simulink model "Step_8_Gravity_compensationController"  (R2020a)
settings: Solver=VariableStepAuto  StartTime=0.0  StopTime=20  FixedStep=1e-3  RelTol=1e-3
values from neighbouring files (symbols this model uses):
  N = simplify(N,'Seconds',30)    [GetTheRegressorMatrix_step1.m]    (also in Step_1_TheRegressorModel.m)
  s = size(M)    [GetTheRegressorMatrix_step1.m]    (also in Step_1_TheRegressorModel.m)
  Y = sym(zeros(robot.nbDOF,numel(Xhi)))    [GetTheRegressorMatrix_step1.m]    (also in Step_1_TheRegressorModel.m)
  Z = robot.symbolicParameters.Z    [GetTheRegressorMatrix_step1.m]    (also in Step_1_TheRegressorModel.m)
undefined symbols (not defined in the file or in its folder): X
libraries: sm_lib x73, nesl_utility x19
(part 1 of 2)
settings Model: Creator=nnnmmm  LastModifiedBy=nnnmmm
settings ExplorerConfigSet: InternalSimMechanicsExplorerSettings="<ExplorerConfiguration><canonicalview>default</canonicalview><AnimationSetting><BasePlaybackSpeed>1.0</BasePlaybackSpeed><PlaybackSpeedFactor>1.0</PlaybackSpeedFactor></AnimationSetting><TilePanel><TileInfo><Tiles Columns=\"1\" Count=\"1\" Rows=\"1\"><Column Weight=\"1\"/><Row Weight=\"1\"/><Tile Height=\"1\" Width=\"1\" X=\"0\" Y=\"0\"/></Tiles></TileInfo><SceneInfo><SceneViewer><BGColor><R>0.60000002384185791</R><G>0.60000002384185791</G><B>0.60000002384185791</B></BGColor><Camera><DoPerspective>off</DoPerspective><Position><X>-0.071417138481595005</X><Y>-0.953379631042480469</Y><Z>-0.0736574933478599397</Z></Position><Center><X>-0.071417138481595005</X><Y>0.0466203689575195104</Y><Z>-0.0736574933478599397</Z></Center><Up><X>0</X><Y>-0</Y><Z>1</Z></Up><ViewLimDist>1</ViewLimDist><YLim>0.662662160254506083</YLim><XLim>1.08174302415975299</XLim></Camera></SceneViewer></SceneInfo></TilePanel><MechEditorPanel><Cameras/><GfxPanelCameraMap/><VideoCreator><PlaybackSpeedRatio>1.0</PlaybackSpeedRatio><FrameRate>60</FrameRate><VideoFormat>MPEG-4</VideoFormat><FrameSize>auto</FrameSize></VideoCreator></MechEditorPanel></ExplorerConfiguration>"

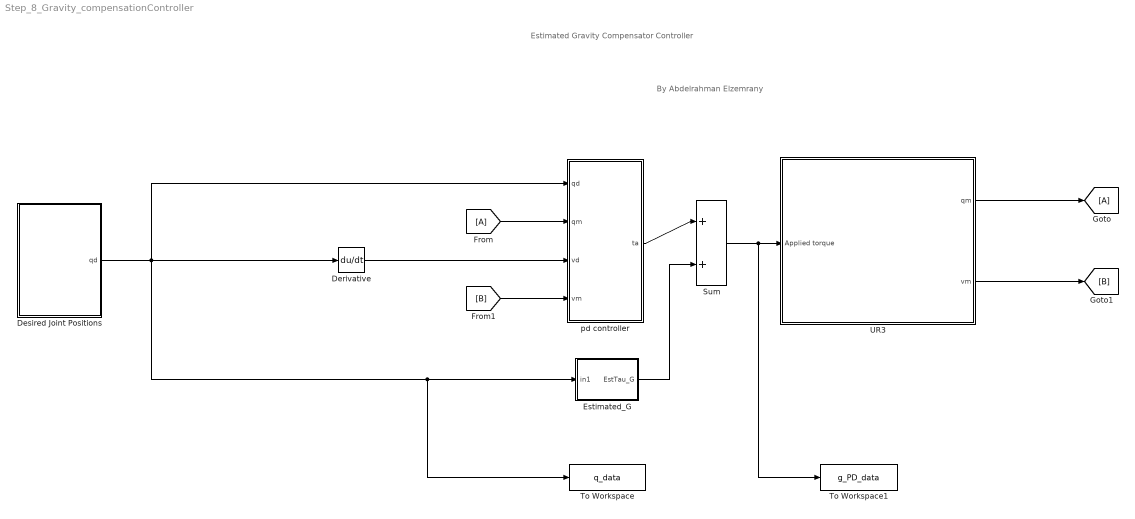
== system Step_8_Gravity_compensationController ==
  note: By Abdelrahman Elzemrany
  note: Estimated Gravity Compensator Controller
  Derivative : Derivative
  Desired Joint Positions : Subsystem
  Estimated_G : MATLAB Function  TreatAsAtomicUnit=on
  Sum : Sum  Inputs=|++
  To Workspace : ToWorkspace  VariableName=q_data  SaveFormat=Timeseries  SampleTime=-1
  To Workspace1 : ToWorkspace  VariableName=g_PD_data  SaveFormat=Timeseries  SampleTime=-1
  UR3 : Subsystem
  pd controller : Subsystem
  wires:
  Desired Joint Positions/1(qd) -> pd controller/1(qd), To Workspace/1, Estimated_G/1(in1), Derivative/1
  Derivative/1 -> pd controller/3(vd)
  Sum/1 -> To Workspace1/1, UR3/1(Applied torque)
  UR3/1(qm) -> [A]
  UR3/2(vm) -> [B]
  [A] -> pd controller/2(qm)
  [B] -> pd controller/4(vm)
  pd controller/1(ta) -> Sum/1
  Estimated_G/1(EstTau_G) -> Sum/2

== system Step_8_Gravity_compensationController/Desired Joint Positions ==
  Mux : Mux  Inputs=6
  Sine Wave : Sin  Frequency=1.5  SampleTime=0
  Sine Wave1 : Sin  Amplitude=1.3  Frequency=.7  SampleTime=0
  Sine Wave2 : Sin  Amplitude=0  Frequency=.9  SampleTime=0
  Sine Wave3 : Sin  Amplitude=0  SampleTime=0
  Sine Wave4 : Sin  Amplitude=01  SampleTime=0
  Sine Wave5 : Sin  Frequency=2  SampleTime=0
  qd : Outport
  wires:
  Sine Wave2/1 -> Mux/3
  Sine Wave1/1 -> Mux/2
  Sine Wave3/1 -> Mux/4
  Sine Wave5/1 -> Mux/6
  Mux/1 -> qd/1
  Sine Wave/1 -> Mux/1
  Sine Wave4/1 -> Mux/5

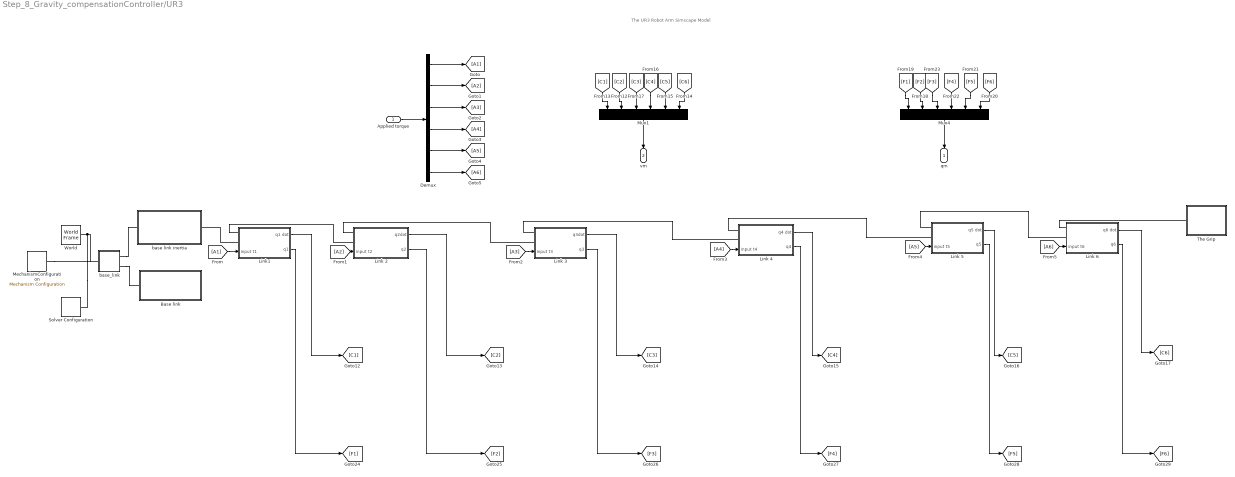
== system Step_8_Gravity_compensationController/UR3 ==
  note: The UR3 Robot Arm Simscape Model
  Applied torque : Inport
  Base link : Subsystem
  Demux : Demux  Outputs=6
  Link 2 : Subsystem
      settings: PortSchema="{\"entries\":[{\"content\":{\"sides\":[{\"content\":{\"connectorIds\":[\"LConn1\",\"LConn2\",\"In1\"]},\"type\":\"ConnectorPlacement.EquallySpacedRectSide\",\"uuid\":\"5cbd8a4c-d881-4795-ab9f-16a1f0c0f3ab\"},{\"content\":{\"connectorIds\":[\"Out1\",\"Out2\"],\"side\":\"RIGHT\"},\"type\":\"ConnectorPlacement.EquallySpacedRectSide\",\"uuid\":\"debf20a3-1058-4606-a7af-87a1301ab1e8\"},{\"content\":{\"connectorIds\":[],\"side\":\"TOP\"},\"type\":\"ConnectorPlacement.EquallySpacedRectSide\",\"uuid\":\"2beda80e-898b-4bea-a963-fb4d7f97ccb8\"}]},\"type\":\"ConnectorPlacement.EquallySpacedConnector\",\"uuid\":\"5c7e1622-356a-471c-9dee-e59231d833b5\"}],\"packageUris\":[\"http://schema.mathworks.com/mf0/Connector/19700101\"],\"version\":\"1.0\"}"
  Link 3 : Subsystem
      settings: PortSchema="{\"entries\":[{\"content\":{\"sides\":[{\"content\":{\"connectorIds\":[\"LConn1\",\"LConn2\",\"In1\"]},\"type\":\"ConnectorPlacement.EquallySpacedRectSide\",\"uuid\":\"5cbd8a4c-d881-4795-ab9f-16a1f0c0f3ab\"},{\"content\":{\"connectorIds\":[\"Out1\",\"Out2\"],\"side\":\"RIGHT\"},\"type\":\"ConnectorPlacement.EquallySpacedRectSide\",\"uuid\":\"debf20a3-1058-4606-a7af-87a1301ab1e8\"},{\"content\":{\"connectorIds\":[],\"side\":\"TOP\"},\"type\":\"ConnectorPlacement.EquallySpacedRectSide\",\"uuid\":\"2beda80e-898b-4bea-a963-fb4d7f97ccb8\"}]},\"type\":\"ConnectorPlacement.EquallySpacedConnector\",\"uuid\":\"5c7e1622-356a-471c-9dee-e59231d833b5\"}],\"packageUris\":[\"http://schema.mathworks.com/mf0/Connector/19700101\"],\"version\":\"1.0\"}"
  Link 4 : Subsystem
      settings: PortSchema="{\"entries\":[{\"content\":{\"sides\":[{\"content\":{\"connectorIds\":[\"LConn1\",\"LConn2\",\"In1\"]},\"type\":\"ConnectorPlacement.EquallySpacedRectSide\",\"uuid\":\"5cbd8a4c-d881-4795-ab9f-16a1f0c0f3ab\"},{\"content\":{\"connectorIds\":[\"Out1\",\"Out2\"],\"side\":\"RIGHT\"},\"type\":\"ConnectorPlacement.EquallySpacedRectSide\",\"uuid\":\"debf20a3-1058-4606-a7af-87a1301ab1e8\"},{\"content\":{\"connectorIds\":[],\"side\":\"TOP\"},\"type\":\"ConnectorPlacement.EquallySpacedRectSide\",\"uuid\":\"2beda80e-898b-4bea-a963-fb4d7f97ccb8\"}]},\"type\":\"ConnectorPlacement.EquallySpacedConnector\",\"uuid\":\"5c7e1622-356a-471c-9dee-e59231d833b5\"}],\"packageUris\":[\"http://schema.mathworks.com/mf0/Connector/19700101\"],\"version\":\"1.0\"}"
  Link 5 : Subsystem
      settings: PortSchema="{\"entries\":[{\"content\":{\"sides\":[{\"content\":{\"connectorIds\":[\"LConn1\",\"LConn2\",\"In1\"]},\"type\":\"ConnectorPlacement.EquallySpacedRectSide\",\"uuid\":\"5cbd8a4c-d881-4795-ab9f-16a1f0c0f3ab\"},{\"content\":{\"connectorIds\":[\"Out1\",\"Out2\"],\"side\":\"RIGHT\"},\"type\":\"ConnectorPlacement.EquallySpacedRectSide\",\"uuid\":\"debf20a3-1058-4606-a7af-87a1301ab1e8\"},{\"content\":{\"connectorIds\":[],\"side\":\"TOP\"},\"type\":\"ConnectorPlacement.EquallySpacedRectSide\",\"uuid\":\"2beda80e-898b-4bea-a963-fb4d7f97ccb8\"}]},\"type\":\"ConnectorPlacement.EquallySpacedConnector\",\"uuid\":\"5c7e1622-356a-471c-9dee-e59231d833b5\"}],\"packageUris\":[\"http://schema.mathworks.com/mf0/Connector/19700101\"],\"version\":\"1.0\"}"
  Link 6 : Subsystem
      settings: PortSchema="{\"entries\":[{\"content\":{\"sides\":[{\"content\":{\"connectorIds\":[\"LConn1\",\"LConn2\",\"In1\"]},\"type\":\"ConnectorPlacement.EquallySpacedRectSide\",\"uuid\":\"5cbd8a4c-d881-4795-ab9f-16a1f0c0f3ab\"},{\"content\":{\"connectorIds\":[\"Out1\",\"Out2\"],\"side\":\"RIGHT\"},\"type\":\"ConnectorPlacement.EquallySpacedRectSide\",\"uuid\":\"debf20a3-1058-4606-a7af-87a1301ab1e8\"},{\"content\":{\"connectorIds\":[],\"side\":\"TOP\"},\"type\":\"ConnectorPlacement.EquallySpacedRectSide\",\"uuid\":\"2beda80e-898b-4bea-a963-fb4d7f97ccb8\"}]},\"type\":\"ConnectorPlacement.EquallySpacedConnector\",\"uuid\":\"5c7e1622-356a-471c-9dee-e59231d833b5\"}],\"packageUris\":[\"http://schema.mathworks.com/mf0/Connector/19700101\"],\"version\":\"1.0\"}"
  Link1 : Subsystem
      settings: PortSchema="{\"entries\":[{\"content\":{\"sides\":[{\"content\":{\"connectorIds\":[\"LConn1\",\"LConn2\",\"In1\"]},\"type\":\"ConnectorPlacement.EquallySpacedRectSide\",\"uuid\":\"5cbd8a4c-d881-4795-ab9f-16a1f0c0f3ab\"},{\"content\":{\"connectorIds\":[\"Out1\",\"Out2\"],\"side\":\"RIGHT\"},\"type\":\"ConnectorPlacement.EquallySpacedRectSide\",\"uuid\":\"debf20a3-1058-4606-a7af-87a1301ab1e8\"},{\"content\":{\"connectorIds\":[],\"side\":\"TOP\"},\"type\":\"ConnectorPlacement.EquallySpacedRectSide\",\"uuid\":\"2beda80e-898b-4bea-a963-fb4d7f97ccb8\"}]},\"type\":\"ConnectorPlacement.EquallySpacedConnector\",\"uuid\":\"5c7e1622-356a-471c-9dee-e59231d833b5\"}],\"packageUris\":[\"http://schema.mathworks.com/mf0/Connector/19700101\"],\"version\":\"1.0\"}"
  MechanismConfiguration : sm_lib/Utilities/Mechanism Configuration  UniformGravity=Constant  GravityVector=[0 0 -9.80665]  GravityUnits=m/s^2  LinearizationDelta=0.001
  Mux1 : Mux  Inputs=6
  Mux4 : Mux  Inputs=6
  Solver Configuration : nesl_utility/Solver Configuration  PhysicalDomain=network_engine_domain  SubClassName=solver  LeftPortType=input  RightPortType=generic  Tones=[]  Harmonics=[]  SimulateNoise=off  Profile=off  UseLocalSampling=off  EnableSwitchedLinearOptims=on  FrequencyDomain=off  UseCCode=off  RelTol=0.001  AbsTol=1e-06  MinStep=1e-09  ToWorkspace=off  RevertToSquareIcSolve=off  NumHomotopyIterations=100  PhasorMode=off  PhasorModeNumHarmonics=1  DoDC=off  ResidualTolerance=1e-09  UseLocalSolver=off  LocalSolverChoice=NE_BACKWARD_EULER_ADVANCER  LocalSolverSampleTime=0.001  DoFixedCost=off  MaxNonlinIter=3  MaxModeIter=2  LinearAlgebra=auto  EquationFormulation=NE_TIME_EF  DelaysMemoryBudget=1024  AutomaticFiltering=on  FilteringTimeConstant=0.001  PartitionStorageMethod=AS_NEEDED  PartitionMemoryBudget=1024  PartitionMethod=ROBUST
  The Grip : Subsystem
  World : sm_lib/Frames and Transforms/World Frame
  base link inertia : Subsystem
  base_link : Subsystem
  qm : Outport
  vm : Outport  Port=2
  wires:
  Applied torque/1 -> Demux/1
  Demux/1 -> [A1]
  Demux/2 -> [A2]
  Demux/3 -> [A3]
  Demux/4 -> [A4]
  Demux/5 -> [A5]
  Demux/6 -> [A6]
  [A1] -> Link1/1(input t1)
  [A2] -> Link 2/1(input t2)
  [A3] -> Link 3/1(input t3)
  [A4] -> Link 4/1(input t4)
  [A5] -> Link 5/1(input t5)
  [A6] -> Link 6/1(input t6)
  Link1/1(q1 dot) -> [C1]
  Link 2/1(q2dot) -> [C2]
  Link 3/1(q3dot) -> [C3]
  Link 4/1(q4 dot) -> [C4]
  Link 5/1(q5 dot) -> [C5]
  Link 6/1(q6 dot) -> [C6]
  Link1/2(q1) -> [F1]
  Link 2/2(q2) -> [F2]
  Link 3/2(q3) -> [F3]
  Link 4/2(q4) -> [F4]
  Link 5/2(q5) -> [F5]
  Link 6/2(q6) -> [F6]
  [C1] -> Mux1/1
  [C6] -> Mux1/6
  [C5] -> Mux1/5
  [C4] -> Mux1/4
  [C2] -> Mux1/2
  [C3] -> Mux1/3
  Mux1/1 -> vm/1
  [F1] -> Mux4/1
  [F6] -> Mux4/6
  [F5] -> Mux4/5
  [F4] -> Mux4/4
  [F2] -> Mux4/2
  [F3] -> Mux4/3
  Mux4/1 -> qm/1
  connections:
  World/RConn1 -- MechanismConfiguration/RConn1 -- Solver Configuration/RConn1 -- base_link/LConn1
  base_link/RConn2 -- Base link/LConn1
  base_link/RConn1 -- base link inertia/LConn1
  Link1/LConn2 -- base link inertia/RConn1
  Link 2/LConn2 -- Link1/LConn1
  Link 3/LConn2 -- Link 2/LConn1
  Link 3/LConn1 -- Link 4/LConn2
  Link 4/LConn1 -- Link 5/LConn2
  Link 5/LConn1 -- Link 6/LConn2
  The Grip/LConn1 -- Link 6/LConn1

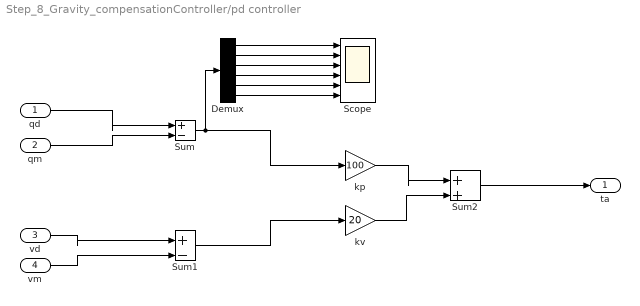
== system Step_8_Gravity_compensationController/pd controller ==
  qd : Inport
  qm : Inport  Port=2
  vd : Inport  Port=3
  vm : Inport  Port=4
  Demux : Demux  Outputs=6
  Scope : Scope  NumInputPorts=6
  Sum : Sum  Inputs=|+-
  Sum1 : Sum  Inputs=|+-
  Sum2 : Sum  Inputs=|++
  kp : Gain  Gain=100
  kv : Gain  Gain=20
  ta : Outport
  wires:
  kp/1 -> Sum2/1
  kv/1 -> Sum2/2
  Sum1/1 -> kv/1
  Sum/1 -> Demux/1, kp/1
  vm/1 -> Sum1/2
  vd/1 -> Sum1/1
  qd/1 -> Sum/1
  qm/1 -> Sum/2
  Sum2/1 -> ta/1
  Demux/1 -> Scope/1
  Demux/2 -> Scope/2
  Demux/3 -> Scope/3
  Demux/4 -> Scope/4
  Demux/5 -> Scope/5
  Demux/6 -> Scope/6

== system Step_8_Gravity_compensationController/UR3/Base link ==
  base : Subsystem
  base_link_base_fixed_joint : sm_lib/Joints/Weld Joint  JointMode=Normal  SenseConstraintForce=off  SenseConstraintForceX=off  SenseConstraintForceY=off  SenseConstraintForceZ=off  SenseConstraintTorque=off  SenseConstraintTorqueX=off  SenseConstraintTorqueY=off  SenseConstraintTorqueZ=off  SenseTotalForce=off  SenseTotalForceX=off  SenseTotalForceY=off  SenseTotalForceZ=off  SenseTotalTorque=off  SenseTotalTorqueX=off  SenseTotalTorqueY=off  SenseTotalTorqueZ=off  CompositeWrenchDir=FollowerOnBase  CompositeWrenchFrame=BaseFrame
  base_link_base_fixed_joint1 : PMIOPort  Side=Left
  connections:
  base/LConn1 -- base_link_base_fixed_joint/RConn1
  base_link_base_fixed_joint1/RConn1 -- base_link_base_fixed_joint/LConn1

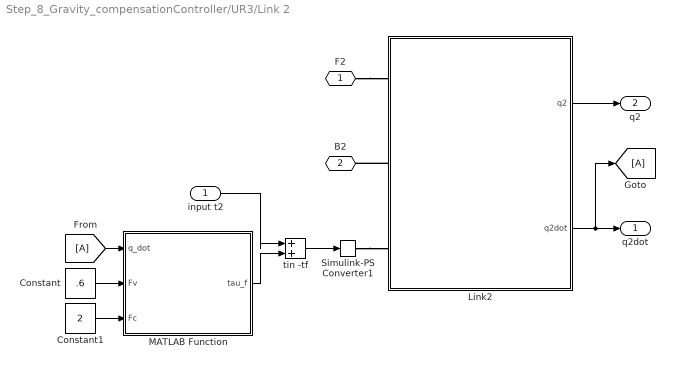
== system Step_8_Gravity_compensationController/UR3/Link 2 ==
  input t2 : Inport
  Constant : Constant  Value=.6
  Constant1 : Constant  Value=2
  Link2 : Subsystem
  MATLAB Function : MATLAB Function  TreatAsAtomicUnit=on
  Simulink-PS Converter1 : nesl_utility/Simulink-PS Converter  PhysicalDomain=network_engine_domain  SubClassName=ps_input  LeftPortType=input  RightPortType=output  PseudoPeriodic=off  Frequencies=[]  NoiseDistribution=none  NoiseParameters=[]  Unit=1  AffineConversion=off  FilteringAndDerivatives=provide  SimscapeFilterOrder=1  InputFilterTimeConstant=0.001  UdotUserProvided=0
  tin -tf : Sum  Inputs=|++
  F2 : PMIOPort  Side=Left
  B2 : PMIOPort  Port=2  Side=Left
  q2dot : Outport
  q2 : Outport  Port=2
  wires:
  Link2/2(q2dot) -> [A], q2dot/1
  Link2/1(q2) -> q2/1
  Constant1/1 -> MATLAB Function/3(Fc)
  MATLAB Function/1(tau_f) -> tin -tf/2
  Constant/1 -> MATLAB Function/2(Fv)
  input t2/1 -> tin -tf/1
  tin -tf/1 -> Simulink-PS Converter1/1
  [A] -> MATLAB Function/1(q_dot)
  connections:
  Simulink-PS Converter1/RConn1 -- Link2/LConn3
  F2/RConn1 -- Link2/LConn1
  Link2/LConn2 -- B2/RConn1

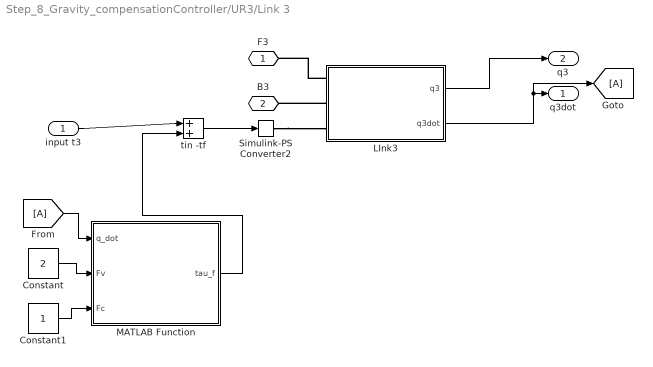
== system Step_8_Gravity_compensationController/UR3/Link 3 ==
  input t3 : Inport
  Constant : Constant  Value=2
  Constant1 : Constant
  LInk3 : Subsystem
  MATLAB Function : MATLAB Function  TreatAsAtomicUnit=on
  Simulink-PS Converter2 : nesl_utility/Simulink-PS Converter  PhysicalDomain=network_engine_domain  SubClassName=ps_input  LeftPortType=input  RightPortType=output  PseudoPeriodic=off  Frequencies=[]  NoiseDistribution=none  NoiseParameters=[]  Unit=1  AffineConversion=off  FilteringAndDerivatives=provide  SimscapeFilterOrder=1  InputFilterTimeConstant=0.001  UdotUserProvided=0
  tin -tf : Sum  Inputs=|++
  F3 : PMIOPort  Side=Left
  B3 : PMIOPort  Port=2  Side=Left
  q3dot : Outport
  q3 : Outport  Port=2
  wires:
  LInk3/1(q3) -> q3/1
  Constant1/1 -> MATLAB Function/3(Fc)
  MATLAB Function/1(tau_f) -> tin -tf/2
  Constant/1 -> MATLAB Function/2(Fv)
  input t3/1 -> tin -tf/1
  tin -tf/1 -> Simulink-PS Converter2/1
  LInk3/2(q3dot) -> [A], q3dot/1
  [A] -> MATLAB Function/1(q_dot)
  connections:
  Simulink-PS Converter2/RConn1 -- LInk3/LConn3
  LInk3/LConn2 -- B3/RConn1
  LInk3/LConn1 -- F3/RConn1

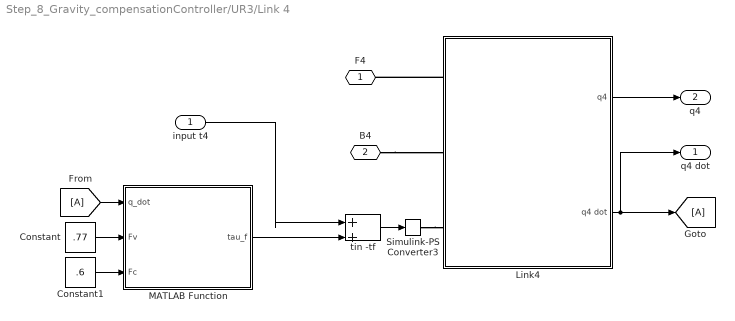
== system Step_8_Gravity_compensationController/UR3/Link 4 ==
  input t4 : Inport
  Constant : Constant  Value=.77
  Constant1 : Constant  Value=.6
  Link4 : Subsystem
  MATLAB Function : MATLAB Function  TreatAsAtomicUnit=on
  Simulink-PS Converter3 : nesl_utility/Simulink-PS Converter  PhysicalDomain=network_engine_domain  SubClassName=ps_input  LeftPortType=input  RightPortType=output  PseudoPeriodic=off  Frequencies=[]  NoiseDistribution=none  NoiseParameters=[]  Unit=1  AffineConversion=off  FilteringAndDerivatives=provide  SimscapeFilterOrder=1  InputFilterTimeConstant=0.001  UdotUserProvided=0
  tin -tf : Sum  Inputs=|++
  F4 : PMIOPort  Side=Left
  B4 : PMIOPort  Port=2  Side=Left
  q4 dot : Outport
  q4 : Outport  Port=2
  wires:
  Link4/1(q4) -> q4/1
  Link4/2(q4 dot) -> q4 dot/1, [A]
  Constant1/1 -> MATLAB Function/3(Fc)
  MATLAB Function/1(tau_f) -> tin -tf/2
  Constant/1 -> MATLAB Function/2(Fv)
  tin -tf/1 -> Simulink-PS Converter3/1
  input t4/1 -> tin -tf/1
  [A] -> MATLAB Function/1(q_dot)
  connections:
  Simulink-PS Converter3/RConn1 -- Link4/LConn3
  B4/RConn1 -- Link4/LConn2
  Link4/LConn1 -- F4/RConn1

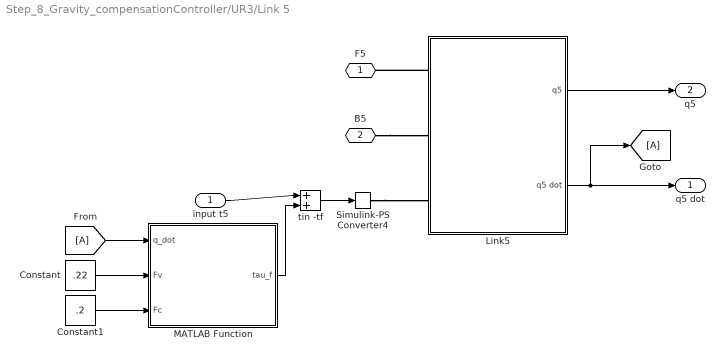
== system Step_8_Gravity_compensationController/UR3/Link 5 ==
  input t5 : Inport
  Constant : Constant  Value=.22
  Constant1 : Constant  Value=.2
  Link5 : Subsystem
  MATLAB Function : MATLAB Function  TreatAsAtomicUnit=on
  Simulink-PS Converter4 : nesl_utility/Simulink-PS Converter  PhysicalDomain=network_engine_domain  SubClassName=ps_input  LeftPortType=input  RightPortType=output  PseudoPeriodic=off  Frequencies=[]  NoiseDistribution=none  NoiseParameters=[]  Unit=1  AffineConversion=off  FilteringAndDerivatives=provide  SimscapeFilterOrder=1  InputFilterTimeConstant=0.001  UdotUserProvided=0
  tin -tf : Sum  Inputs=|++
  F5 : PMIOPort  Side=Left
  B5 : PMIOPort  Port=2  Side=Left
  q5 dot : Outport
  q5 : Outport  Port=2
  wires:
  Link5/1(q5) -> q5/1
  Link5/2(q5 dot) -> [A], q5 dot/1
  Constant1/1 -> MATLAB Function/3(Fc)
  MATLAB Function/1(tau_f) -> tin -tf/2
  Constant/1 -> MATLAB Function/2(Fv)
  input t5/1 -> tin -tf/1
  tin -tf/1 -> Simulink-PS Converter4/1
  [A] -> MATLAB Function/1(q_dot)
  connections:
  Simulink-PS Converter4/RConn1 -- Link5/LConn3
  B5/RConn1 -- Link5/LConn2
  Link5/LConn1 -- F5/RConn1

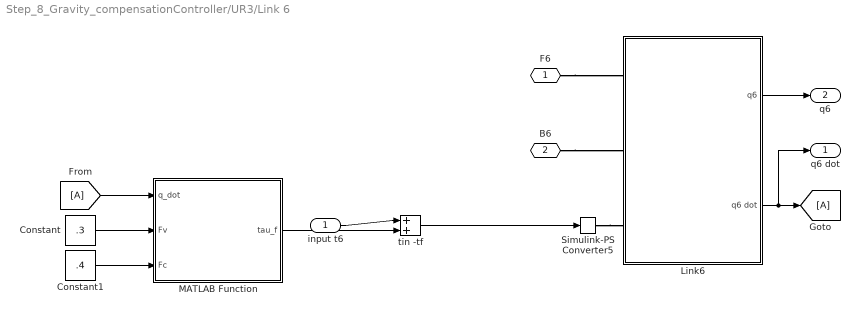
== system Step_8_Gravity_compensationController/UR3/Link 6 ==
  input t6 : Inport
  Constant : Constant  Value=.3
  Constant1 : Constant  Value=.4
  Link6 : Subsystem
  MATLAB Function : MATLAB Function  TreatAsAtomicUnit=on
  Simulink-PS Converter5 : nesl_utility/Simulink-PS Converter  PhysicalDomain=network_engine_domain  SubClassName=ps_input  LeftPortType=input  RightPortType=output  PseudoPeriodic=off  Frequencies=[]  NoiseDistribution=none  NoiseParameters=[]  Unit=1  AffineConversion=off  FilteringAndDerivatives=provide  SimscapeFilterOrder=1  InputFilterTimeConstant=0.001  UdotUserProvided=0
  tin -tf : Sum  Inputs=|++
  F6 : PMIOPort  Side=Left
  B6 : PMIOPort  Port=2  Side=Left
  q6 dot : Outport
  q6 : Outport  Port=2
  wires:
  Link6/1(q6) -> q6/1
  Link6/2(q6 dot) -> q6 dot/1, [A]
  Constant1/1 -> MATLAB Function/3(Fc)
  MATLAB Function/1(tau_f) -> tin -tf/2
  Constant/1 -> MATLAB Function/2(Fv)
  input t6/1 -> tin -tf/1
  tin -tf/1 -> Simulink-PS Converter5/1
  [A] -> MATLAB Function/1(q_dot)
  connections:
  Simulink-PS Converter5/RConn1 -- Link6/LConn3
  F6/RConn1 -- Link6/LConn1
  B6/RConn1 -- Link6/LConn2

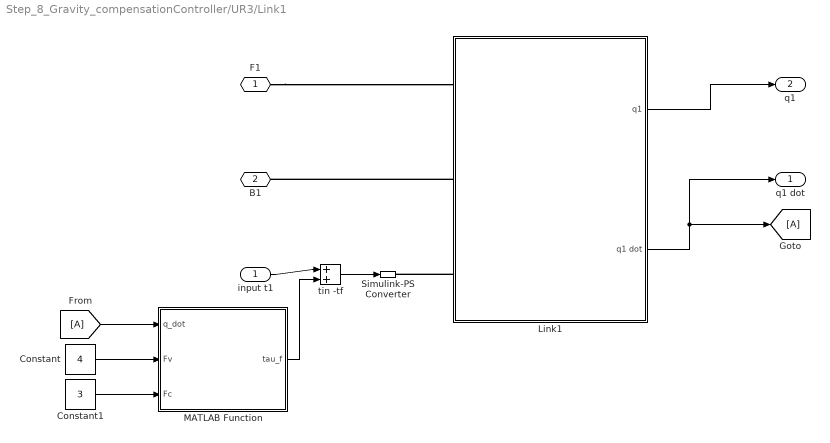
== system Step_8_Gravity_compensationController/UR3/Link1 ==
  input t1 : Inport
  Constant : Constant  Value=4
  Constant1 : Constant  Value=3
  Link1 : Subsystem
  MATLAB Function : MATLAB Function  TreatAsAtomicUnit=on
  Simulink-PS Converter : nesl_utility/Simulink-PS Converter  PhysicalDomain=network_engine_domain  SubClassName=ps_input  LeftPortType=input  RightPortType=output  PseudoPeriodic=off  Frequencies=[]  NoiseDistribution=none  NoiseParameters=[]  Unit=1  AffineConversion=off  FilteringAndDerivatives=provide  SimscapeFilterOrder=1  InputFilterTimeConstant=0.001  UdotUserProvided=0
  tin -tf : Sum  Inputs=|++
  F1 : PMIOPort  Side=Left
  B1 : PMIOPort  Port=2  Side=Left
  q1 dot : Outport
  q1 : Outport  Port=2
  wires:
  Link1/1(q1) -> q1/1
  Link1/2(q1 dot) -> q1 dot/1, [A]
  input t1/1 -> tin -tf/1
  tin -tf/1 -> Simulink-PS Converter/1
  MATLAB Function/1(tau_f) -> tin -tf/2
  Constant/1 -> MATLAB Function/2(Fv)
  Constant1/1 -> MATLAB Function/3(Fc)
  [A] -> MATLAB Function/1(q_dot)
  connections:
  Link1/LConn2 -- B1/RConn1
  Link1/LConn3 -- Simulink-PS Converter/RConn1
  F1/RConn1 -- Link1/LConn1

== system Step_8_Gravity_compensationController/UR3/The Grip ==
  flange : Subsystem
  flange_tool0 : sm_lib/Joints/Weld Joint  JointMode=Normal  SenseConstraintForce=off  SenseConstraintForceX=off  SenseConstraintForceY=off  SenseConstraintForceZ=off  SenseConstraintTorque=off  SenseConstraintTorqueX=off  SenseConstraintTorqueY=off  SenseConstraintTorqueZ=off  SenseTotalForce=off  SenseTotalForceX=off  SenseTotalForceY=off  SenseTotalForceZ=off  SenseTotalTorque=off  SenseTotalTorqueX=off  SenseTotalTorqueY=off  SenseTotalTorqueZ=off  CompositeWrenchDir=FollowerOnBase  CompositeWrenchFrame=BaseFrame
  tool0 : Subsystem
  wrist_3_flange : sm_lib/Joints/Weld Joint  JointMode=Normal  SenseConstraintForce=off  SenseConstraintForceX=off  SenseConstraintForceY=off  SenseConstraintForceZ=off  SenseConstraintTorque=off  SenseConstraintTorqueX=off  SenseConstraintTorqueY=off  SenseConstraintTorqueZ=off  SenseTotalForce=off  SenseTotalForceX=off  SenseTotalForceY=off  SenseTotalForceZ=off  SenseTotalTorque=off  SenseTotalTorqueX=off  SenseTotalTorqueY=off  SenseTotalTorqueZ=off  CompositeWrenchDir=FollowerOnBase  CompositeWrenchFrame=BaseFrame
  wrist_3_flange1 : PMIOPort  Side=Left
  connections:
  flange/LConn1 -- wrist_3_flange/RConn1
  flange_tool0/RConn1 -- tool0/LConn1
  flange/RConn1 -- flange_tool0/LConn1
  wrist_3_flange/LConn1 -- wrist_3_flange1/RConn1

== system Step_8_Gravity_compensationController/UR3/base link inertia ==
  base_link_base_link_inertia : sm_lib/Joints/Weld Joint  JointMode=Normal  SenseConstraintForce=off  SenseConstraintForceX=off  SenseConstraintForceY=off  SenseConstraintForceZ=off  SenseConstraintTorque=off  SenseConstraintTorqueX=off  SenseConstraintTorqueY=off  SenseConstraintTorqueZ=off  SenseTotalForce=off  SenseTotalForceX=off  SenseTotalForceY=off  SenseTotalForceZ=off  SenseTotalTorque=off  SenseTotalTorqueX=off  SenseTotalTorqueY=off  SenseTotalTorqueZ=off  CompositeWrenchDir=FollowerOnBase  CompositeWrenchFrame=BaseFrame
  base_link_inertia : Subsystem
  F1 : PMIOPort  Side=Right
  base_link_base_link_inertia1 : PMIOPort  Port=2  Side=Left
  connections:
  base_link_base_link_inertia/RConn1 -- base_link_inertia/LConn1
  base_link_base_link_inertia1/RConn1 -- base_link_base_link_inertia/LConn1
  F1/RConn1 -- base_link_inertia/RConn1

== system Step_8_Gravity_compensationController/UR3/base_link ==
  ReferenceFrame : sm_lib/Frames and Transforms/Reference Frame
  base_link_base_fixed_joint_OriginTransform : sm_lib/Frames and Transforms/Rigid Transform  TranslationMethod=Cartesian  TranslationStandardOffset=0  TranslationLengthUnit=m  TranslationStandardAxis=+Z  TranslationCartesianOffset=[0, 0, 0]  TranslationROffset=0  TranslationROffsetUnits=m  TranslationZOffset=0  TranslationZOffsetUnits=m  TranslationThetaOffset=0  TranslationThetaOffsetUnits=deg  RotationMethod=RotationSequence  RotationAngleUnits=deg  RotationStandardAxis=+Z  RotationAngle=0.0  RotationArbitraryAxis=[0 0 1]  FollAlignAxisA=+X  BaseAlignAxisA=+Y  FollAlignAxisB=+Y  BaseAlignAxisB=+Z  RotationSequenceAxes=BaseAxes  RotationSequence=XYZ  RotationSequenceAngles=[0, 0, 3.141592653589793]  RotationSequenceAnglesUnits=rad  RotationMatrix=[1 0 0; 0 1 0; 0 0 1]
  base_link_base_link_inertia_OriginTransform : sm_lib/Frames and Transforms/Rigid Transform  TranslationMethod=Cartesian  TranslationStandardOffset=0  TranslationLengthUnit=m  TranslationStandardAxis=+Z  TranslationCartesianOffset=[0, 0, 0]  TranslationROffset=0  TranslationROffsetUnits=m  TranslationZOffset=0  TranslationZOffsetUnits=m  TranslationThetaOffset=0  TranslationThetaOffsetUnits=deg  RotationMethod=RotationSequence  RotationAngleUnits=deg  RotationStandardAxis=+Z  RotationAngle=0.0  RotationArbitraryAxis=[0 0 1]  FollAlignAxisA=+X  BaseAlignAxisA=+Y  FollAlignAxisB=+Y  BaseAlignAxisB=+Z  RotationSequenceAxes=BaseAxes  RotationSequence=XYZ  RotationSequenceAngles=[0, 0, 3.141592653589793]  RotationSequenceAnglesUnits=rad  RotationMatrix=[1 0 0; 0 1 0; 0 0 1]
  F : PMIOPort  Side=Left
  F2 : PMIOPort  Port=2  Side=Right
  F1 : PMIOPort  Port=3  Side=Right
  connections:
  base_link_base_fixed_joint_OriginTransform/LConn1 -- ReferenceFrame/RConn1 -- F/RConn1 -- base_link_base_link_inertia_OriginTransform/LConn1
  base_link_base_fixed_joint_OriginTransform/RConn1 -- F1/RConn1
  base_link_base_link_inertia_OriginTransform/RConn1 -- F2/RConn1

== system Step_8_Gravity_compensationController/UR3/Base link/base ==
  ReferenceFrame : sm_lib/Frames and Transforms/Reference Frame
  F : PMIOPort  Side=Left
  connections:
  ReferenceFrame/RConn1 -- F/RConn1

== system Step_8_Gravity_compensationController/UR3/Link 2/Link2 ==
  PS-Simulink Converter5 : nesl_utility/PS-Simulink Converter  PhysicalDomain=network_engine_domain  SubClassName=ps_output  LeftPortType=input  RightPortType=output  PseudoPeriodic=off  Frequencies=[]  Unit=inherit  AffineConversion=off
  PS-Simulink Converter8 : nesl_utility/PS-Simulink Converter  PhysicalDomain=network_engine_domain  SubClassName=ps_output  LeftPortType=input  RightPortType=output  PseudoPeriodic=off  Frequencies=[]  Unit=inherit  AffineConversion=off
  shoulder_lift_joint : sm_lib/Joints/Revolute Joint  JointMode=Normal  SenseConstraintForce=off  SenseConstraintForceX=off  SenseConstraintForceY=off  SenseConstraintForceZ=off  SenseConstraintTorque=off  SenseConstraintTorqueX=off  SenseConstraintTorqueY=off  SenseConstraintTorqueZ=off  SenseTotalForce=off  SenseTotalForceX=off  SenseTotalForceY=off  SenseTotalForceZ=off  SenseTotalTorque=off  SenseTotalTorqueX=off  SenseTotalTorqueY=off  SenseTotalTorqueZ=off  CompositeWrenchDir=FollowerOnBase  CompositeWrenchFrame=BaseFrame  EquilibriumPosition=0  EquilibriumPositionUnits=deg  SpringStiffness=0  SpringStiffnessUnits=N*m/deg  DampingCoefficient=0  DampingCoefficientUnits=m^2*kg/s/rad  TorqueActuationMode=InputTorque  MotionActuationMode=ComputedMotion  SensePosition=on  SenseVelocity=on  SenseAcceleration=off  SenseTorqueForce=off  SenseLowerLimitTorqueForce=off  SenseUpperLimitTorqueForce=off  LowerLimitSpecify=on  LowerLimitBound=-6.283185307179586  LowerLimitBoundUnits=rad  LowerLimitStiffness=1e4  LowerLimitStiffnessUnits=N*m/deg  LowerLimitDamping=10  LowerLimitDampingUnits=N*m/(deg/s)  LowerLimitTransitionRegionWidth=0.1  LowerLimitTransitionRegionWidthUnits=deg  UpperLimitSpecify=on  UpperLimitBound=6.283185307179586  UpperLimitBoundUnits=rad  UpperLimitStiffness=1e4  UpperLimitStiffnessUnits=N*m/deg  UpperLimitDamping=10  UpperLimitDampingUnits=N*m/(deg/s)  UpperLimitTransitionRegionWidth=0.1  UpperLimitTransitionRegionWidthUnits=deg  PositionTargetSpecify=off  PositionTargetPriority=High  PositionTargetValue=0  PositionTargetValueUnits=deg  VelocityTargetSpecify=off  VelocityTargetPriority=High  VelocityTargetValue=0  VelocityTargetValueUnits=deg/s
  upper_arm_link : Subsystem
  F1 : PMIOPort  Side=Left
  B2 : PMIOPort  Port=2  Side=Left
  t2 : PMIOPort  Port=3  Side=Left
  q2 : Outport
  q2dot : Outport  Port=2
  wires:
  PS-Simulink Converter5/1 -> q2/1
  PS-Simulink Converter8/1 -> q2dot/1
  connections:
  shoulder_lift_joint/RConn1 -- upper_arm_link/LConn1
  F1/RConn1 -- upper_arm_link/RConn1
  shoulder_lift_joint/LConn1 -- B2/RConn1
  t2/RConn1 -- shoulder_lift_joint/LConn2
  shoulder_lift_joint/RConn3 -- PS-Simulink Converter8/LConn1
  shoulder_lift_joint/RConn2 -- PS-Simulink Converter5/LConn1

== system Step_8_Gravity_compensationController/UR3/Link 3/LInk3 ==
  PS-Simulink Converter2 : nesl_utility/PS-Simulink Converter  PhysicalDomain=network_engine_domain  SubClassName=ps_output  LeftPortType=input  RightPortType=output  PseudoPeriodic=off  Frequencies=[]  Unit=inherit  AffineConversion=off
  PS-Simulink Converter7 : nesl_utility/PS-Simulink Converter  PhysicalDomain=network_engine_domain  SubClassName=ps_output  LeftPortType=input  RightPortType=output  PseudoPeriodic=off  Frequencies=[]  Unit=inherit  AffineConversion=off
  elbow_joint : sm_lib/Joints/Revolute Joint  JointMode=Normal  SenseConstraintForce=off  SenseConstraintForceX=off  SenseConstraintForceY=off  SenseConstraintForceZ=off  SenseConstraintTorque=off  SenseConstraintTorqueX=off  SenseConstraintTorqueY=off  SenseConstraintTorqueZ=off  SenseTotalForce=off  SenseTotalForceX=off  SenseTotalForceY=off  SenseTotalForceZ=off  SenseTotalTorque=off  SenseTotalTorqueX=off  SenseTotalTorqueY=off  SenseTotalTorqueZ=off  CompositeWrenchDir=FollowerOnBase  CompositeWrenchFrame=BaseFrame  EquilibriumPosition=0  EquilibriumPositionUnits=deg  SpringStiffness=0  SpringStiffnessUnits=N*m/deg  DampingCoefficient=0  DampingCoefficientUnits=m^2*kg/s/rad  TorqueActuationMode=InputTorque  MotionActuationMode=ComputedMotion  SensePosition=on  SenseVelocity=on  SenseAcceleration=off  SenseTorqueForce=off  SenseLowerLimitTorqueForce=off  SenseUpperLimitTorqueForce=off  LowerLimitSpecify=on  LowerLimitBound=-3.141592653589793  LowerLimitBoundUnits=rad  LowerLimitStiffness=1e4  LowerLimitStiffnessUnits=N*m/deg  LowerLimitDamping=10  LowerLimitDampingUnits=N*m/(deg/s)  LowerLimitTransitionRegionWidth=0.1  LowerLimitTransitionRegionWidthUnits=deg  UpperLimitSpecify=on  UpperLimitBound=3.141592653589793  UpperLimitBoundUnits=rad  UpperLimitStiffness=1e4  UpperLimitStiffnessUnits=N*m/deg  UpperLimitDamping=10  UpperLimitDampingUnits=N*m/(deg/s)  UpperLimitTransitionRegionWidth=0.1  UpperLimitTransitionRegionWidthUnits=deg  PositionTargetSpecify=off  PositionTargetPriority=High  PositionTargetValue=0  PositionTargetValueUnits=deg  VelocityTargetSpecify=off  VelocityTargetPriority=High  VelocityTargetValue=0  VelocityTargetValueUnits=deg/s
  forearm_link : Subsystem
  F3 : PMIOPort  Side=Left
  B3 : PMIOPort  Port=2  Side=Left
  t3 : PMIOPort  Port=3  Side=Left
  q3 : Outport
  q3dot : Outport  Port=2
  wires:
  PS-Simulink Converter7/1 -> q3dot/1
  PS-Simulink Converter2/1 -> q3/1
  connections:
  elbow_joint/RConn3 -- PS-Simulink Converter7/LConn1
  t3/RConn1 -- elbow_joint/LConn2
  elbow_joint/LConn1 -- B3/RConn1
  elbow_joint/RConn1 -- forearm_link/LConn1
  elbow_joint/RConn2 -- PS-Simulink Converter2/LConn1
  forearm_link/RConn1 -- F3/RConn1

== system Step_8_Gravity_compensationController/UR3/Link 4/Link4 ==
  PS-Simulink Converter10 : nesl_utility/PS-Simulink Converter  PhysicalDomain=network_engine_domain  SubClassName=ps_output  LeftPortType=input  RightPortType=output  PseudoPeriodic=off  Frequencies=[]  Unit=inherit  AffineConversion=off
  PS-Simulink Converter3 : nesl_utility/PS-Simulink Converter  PhysicalDomain=network_engine_domain  SubClassName=ps_output  LeftPortType=input  RightPortType=output  PseudoPeriodic=off  Frequencies=[]  Unit=inherit  AffineConversion=off
  wrist_1_joint : sm_lib/Joints/Revolute Joint  JointMode=Normal  SenseConstraintForce=off  SenseConstraintForceX=off  SenseConstraintForceY=off  SenseConstraintForceZ=off  SenseConstraintTorque=off  SenseConstraintTorqueX=off  SenseConstraintTorqueY=off  SenseConstraintTorqueZ=off  SenseTotalForce=off  SenseTotalForceX=off  SenseTotalForceY=off  SenseTotalForceZ=off  SenseTotalTorque=off  SenseTotalTorqueX=off  SenseTotalTorqueY=off  SenseTotalTorqueZ=off  CompositeWrenchDir=FollowerOnBase  CompositeWrenchFrame=BaseFrame  EquilibriumPosition=0  EquilibriumPositionUnits=deg  SpringStiffness=0  SpringStiffnessUnits=N*m/deg  DampingCoefficient=0  DampingCoefficientUnits=m^2*kg/s/rad  TorqueActuationMode=InputTorque  MotionActuationMode=ComputedMotion  SensePosition=on  SenseVelocity=on  SenseAcceleration=off  SenseTorqueForce=off  SenseLowerLimitTorqueForce=off  SenseUpperLimitTorqueForce=off  LowerLimitSpecify=on  LowerLimitBound=-6.283185307179586  LowerLimitBoundUnits=rad  LowerLimitStiffness=1e4  LowerLimitStiffnessUnits=N*m/deg  LowerLimitDamping=10  LowerLimitDampingUnits=N*m/(deg/s)  LowerLimitTransitionRegionWidth=0.1  LowerLimitTransitionRegionWidthUnits=deg  UpperLimitSpecify=on  UpperLimitBound=6.283185307179586  UpperLimitBoundUnits=rad  UpperLimitStiffness=1e4  UpperLimitStiffnessUnits=N*m/deg  UpperLimitDamping=10  UpperLimitDampingUnits=N*m/(deg/s)  UpperLimitTransitionRegionWidth=0.1  UpperLimitTransitionRegionWidthUnits=deg  PositionTargetSpecify=off  PositionTargetPriority=High  PositionTargetValue=0  PositionTargetValueUnits=deg  VelocityTargetSpecify=off  VelocityTargetPriority=High  VelocityTargetValue=0  VelocityTargetValueUnits=deg/s
  wrist_1_link : Subsystem
  F4 : PMIOPort  Side=Left
  B4 : PMIOPort  Port=2  Side=Left
  t4 : PMIOPort  Port=3  Side=Left
  q4 : Outport
  q4 dot : Outport  Port=2
  wires:
  PS-Simulink Converter10/1 -> q4 dot/1
  PS-Simulink Converter3/1 -> q4/1
  connections:
  t4/RConn1 -- wrist_1_joint/LConn2
  wrist_1_joint/RConn3 -- PS-Simulink Converter10/LConn1
  wrist_1_joint/RConn2 -- PS-Simulink Converter3/LConn1
  wrist_1_joint/RConn1 -- wrist_1_link/LConn1
  wrist_1_link/RConn1 -- F4/RConn1
  B4/RConn1 -- wrist_1_joint/LConn1

== system Step_8_Gravity_compensationController/UR3/Link 5/Link5 ==
  PS-Simulink Converter11 : nesl_utility/PS-Simulink Converter  PhysicalDomain=network_engine_domain  SubClassName=ps_output  LeftPortType=input  RightPortType=output  PseudoPeriodic=off  Frequencies=[]  Unit=inherit  AffineConversion=off
  PS-Simulink Converter4 : nesl_utility/PS-Simulink Converter  PhysicalDomain=network_engine_domain  SubClassName=ps_output  LeftPortType=input  RightPortType=output  PseudoPeriodic=off  Frequencies=[]  Unit=inherit  AffineConversion=off
  wrist_2_joint : sm_lib/Joints/Revolute Joint  JointMode=Normal  SenseConstraintForce=off  SenseConstraintForceX=off  SenseConstraintForceY=off  SenseConstraintForceZ=off  SenseConstraintTorque=off  SenseConstraintTorqueX=off  SenseConstraintTorqueY=off  SenseConstraintTorqueZ=off  SenseTotalForce=off  SenseTotalForceX=off  SenseTotalForceY=off  SenseTotalForceZ=off  SenseTotalTorque=off  SenseTotalTorqueX=off  SenseTotalTorqueY=off  SenseTotalTorqueZ=off  CompositeWrenchDir=FollowerOnBase  CompositeWrenchFrame=BaseFrame  EquilibriumPosition=0  EquilibriumPositionUnits=deg  SpringStiffness=0  SpringStiffnessUnits=N*m/deg  DampingCoefficient=0  DampingCoefficientUnits=m^2*kg/s/rad  TorqueActuationMode=InputTorque  MotionActuationMode=ComputedMotion  SensePosition=on  SenseVelocity=on  SenseAcceleration=off  SenseTorqueForce=off  SenseLowerLimitTorqueForce=off  SenseUpperLimitTorqueForce=off  LowerLimitSpecify=on  LowerLimitBound=-6.283185307179586  LowerLimitBoundUnits=rad  LowerLimitStiffness=1e4  LowerLimitStiffnessUnits=N*m/deg  LowerLimitDamping=10  LowerLimitDampingUnits=N*m/(deg/s)  LowerLimitTransitionRegionWidth=0.1  LowerLimitTransitionRegionWidthUnits=deg  UpperLimitSpecify=on  UpperLimitBound=6.283185307179586  UpperLimitBoundUnits=rad  UpperLimitStiffness=1e4  UpperLimitStiffnessUnits=N*m/deg  UpperLimitDamping=10  UpperLimitDampingUnits=N*m/(deg/s)  UpperLimitTransitionRegionWidth=0.1  UpperLimitTransitionRegionWidthUnits=deg  PositionTargetSpecify=off  PositionTargetPriority=High  PositionTargetValue=0  PositionTargetValueUnits=deg  VelocityTargetSpecify=off  VelocityTargetPriority=High  VelocityTargetValue=0  VelocityTargetValueUnits=deg/s
  wrist_2_link : Subsystem
  F5 : PMIOPort  Side=Left
  B5 : PMIOPort  Port=2  Side=Left
  t5 : PMIOPort  Port=3  Side=Left
  q5 : Outport
  q5 dot : Outport  Port=2
  wires:
  PS-Simulink Converter4/1 -> q5/1
  PS-Simulink Converter11/1 -> q5 dot/1
  connections:
  B5/RConn1 -- wrist_2_joint/LConn1
  wrist_2_link/RConn1 -- F5/RConn1
  wrist_2_joint/RConn2 -- PS-Simulink Converter4/LConn1
  wrist_2_joint/RConn3 -- PS-Simulink Converter11/LConn1
  t5/RConn1 -- wrist_2_joint/LConn2
  wrist_2_joint/RConn1 -- wrist_2_link/LConn1

== system Step_8_Gravity_compensationController/UR3/Link 6/Link6 ==
  PS-Simulink Converter12 : nesl_utility/PS-Simulink Converter  PhysicalDomain=network_engine_domain  SubClassName=ps_output  LeftPortType=input  RightPortType=output  PseudoPeriodic=off  Frequencies=[]  Unit=inherit  AffineConversion=off
  PS-Simulink Converter6 : nesl_utility/PS-Simulink Converter  PhysicalDomain=network_engine_domain  SubClassName=ps_output  LeftPortType=input  RightPortType=output  PseudoPeriodic=off  Frequencies=[]  Unit=inherit  AffineConversion=off
  wrist_3_joint : sm_lib/Joints/Revolute Joint  JointMode=Normal  SenseConstraintForce=off  SenseConstraintForceX=off  SenseConstraintForceY=off  SenseConstraintForceZ=off  SenseConstraintTorque=off  SenseConstraintTorqueX=off  SenseConstraintTorqueY=off  SenseConstraintTorqueZ=off  SenseTotalForce=off  SenseTotalForceX=off  SenseTotalForceY=off  SenseTotalForceZ=off  SenseTotalTorque=off  SenseTotalTorqueX=off  SenseTotalTorqueY=off  SenseTotalTorqueZ=off  CompositeWrenchDir=FollowerOnBase  CompositeWrenchFrame=BaseFrame  EquilibriumPosition=0  EquilibriumPositionUnits=deg  SpringStiffness=0  SpringStiffnessUnits=N*m/deg  DampingCoefficient=0  DampingCoefficientUnits=m^2*kg/s/rad  TorqueActuationMode=InputTorque  MotionActuationMode=ComputedMotion  SensePosition=on  SenseVelocity=on  SenseAcceleration=off  SenseTorqueForce=off  SenseLowerLimitTorqueForce=off  SenseUpperLimitTorqueForce=off  LowerLimitSpecify=on  LowerLimitBound=-6.283185307179586  LowerLimitBoundUnits=rad  LowerLimitStiffness=1e4  LowerLimitStiffnessUnits=N*m/deg  LowerLimitDamping=10  LowerLimitDampingUnits=N*m/(deg/s)  LowerLimitTransitionRegionWidth=0.1  LowerLimitTransitionRegionWidthUnits=deg  UpperLimitSpecify=on  UpperLimitBound=6.283185307179586  UpperLimitBoundUnits=rad  UpperLimitStiffness=1e4  UpperLimitStiffnessUnits=N*m/deg  UpperLimitDamping=10  UpperLimitDampingUnits=N*m/(deg/s)  UpperLimitTransitionRegionWidth=0.1  UpperLimitTransitionRegionWidthUnits=deg  PositionTargetSpecify=off  PositionTargetPriority=High  PositionTargetValue=0  PositionTargetValueUnits=deg  VelocityTargetSpecify=off  VelocityTargetPriority=High  VelocityTargetValue=0  VelocityTargetValueUnits=deg/s
  wrist_3_link : Subsystem
  F6 : PMIOPort  Side=Left
  B6 : PMIOPort  Port=2  Side=Left
  t6 : PMIOPort  Port=3  Side=Left
  q6 : Outport
  q6 dot : Outport  Port=2
  wires:
  PS-Simulink Converter12/1 -> q6 dot/1
  PS-Simulink Converter6/1 -> q6/1
  connections:
  wrist_3_joint/RConn3 -- PS-Simulink Converter12/LConn1
  F6/RConn1 -- wrist_3_link/RConn1
  wrist_3_joint/RConn1 -- wrist_3_link/LConn1
  wrist_3_joint/RConn2 -- PS-Simulink Converter6/LConn1
  t6/RConn1 -- wrist_3_joint/LConn2
  B6/RConn1 -- wrist_3_joint/LConn1

== system Step_8_Gravity_compensationController/UR3/Link1/Link1 ==
  PS-Simulink Converter1 : nesl_utility/PS-Simulink Converter  PhysicalDomain=network_engine_domain  SubClassName=ps_output  LeftPortType=input  RightPortType=output  PseudoPeriodic=off  Frequencies=[]  Unit=inherit  AffineConversion=off
  PS-Simulink Converter9 : nesl_utility/PS-Simulink Converter  PhysicalDomain=network_engine_domain  SubClassName=ps_output  LeftPortType=input  RightPortType=output  PseudoPeriodic=off  Frequencies=[]  Unit=inherit  AffineConversion=off
  Subsystem : Subsystem
  F1 : PMIOPort  Side=Left
  B1 : PMIOPort  Port=2  Side=Left
  t1 : PMIOPort  Port=3  Side=Left
  q1 : Outport
  q1 dot : Outport  Port=2
  wires:
  PS-Simulink Converter9/1 -> q1 dot/1
  PS-Simulink Converter1/1 -> q1/1
  connections:
  F1/RConn1 -- Subsystem/RConn1
  Subsystem/RConn2 -- PS-Simulink Converter1/LConn1
  Subsystem/LConn1 -- B1/RConn1
  Subsystem/RConn3 -- PS-Simulink Converter9/LConn1
  Subsystem/LConn2 -- t1/RConn1

== system Step_8_Gravity_compensationController/UR3/The Grip/flange ==
  ReferenceFrame : sm_lib/Frames and Transforms/Reference Frame
  flange_tool0_OriginTransform : sm_lib/Frames and Transforms/Rigid Transform  TranslationMethod=Cartesian  TranslationStandardOffset=0  TranslationLengthUnit=m  TranslationStandardAxis=+Z  TranslationCartesianOffset=[0, 0, 0]  TranslationROffset=0  TranslationROffsetUnits=m  TranslationZOffset=0  TranslationZOffsetUnits=m  TranslationThetaOffset=0  TranslationThetaOffsetUnits=deg  RotationMethod=RotationSequence  RotationAngleUnits=deg  RotationStandardAxis=+Z  RotationAngle=0.0  RotationArbitraryAxis=[0 0 1]  FollAlignAxisA=+X  BaseAlignAxisA=+Y  FollAlignAxisB=+Y  BaseAlignAxisB=+Z  RotationSequenceAxes=BaseAxes  RotationSequence=XYZ  RotationSequenceAngles=[1.570796326794897, 0, 1.570796326794897]  RotationSequenceAnglesUnits=rad  RotationMatrix=[1 0 0; 0 1 0; 0 0 1]
  F : PMIOPort  Side=Left
  F1 : PMIOPort  Port=2  Side=Right
  connections:
  flange_tool0_OriginTransform/LConn1 -- ReferenceFrame/RConn1 -- F/RConn1
  flange_tool0_OriginTransform/RConn1 -- F1/RConn1

== system Step_8_Gravity_compensationController/UR3/The Grip/tool0 ==
  ReferenceFrame : sm_lib/Frames and Transforms/Reference Frame
  F : PMIOPort  Side=Left
  connections:
  ReferenceFrame/RConn1 -- F/RConn1

== system Step_8_Gravity_compensationController/UR3/base link inertia/base_link_inertia ==
  Inertia : sm_lib/Body Elements/Inertia  InertiaType=Custom  Mass=2  MassUnits=kg  CenterOfMass=[0, 0, 0]  CenterOfMassUnits=m  MomentsOfInertia=[0.0030531654454, 0.0030531654454, 0.005625]  MomentsOfInertiaUnits=kg*m^2  ProductsOfInertia=[0, 0, 0]  ProductsOfInertiaUnits=kg*m^2  GraphicType=None  MarkerShape=Inertia  MarkerSize=20  GraphicVisPropType=SimpleVisualProperties  GraphicDiffuseColor=[0.5 0.5 0.5]  GraphicSpecularColor=[0.5 0.5 0.5 1.0]  GraphicAmbientColor=[0.15 0.15 0.15 1.0]  GraphicEmissiveColor=[0.0 0.0 0.0 1.0]  GraphicShininess=75  GraphicOpacity=1.0
  InertiaOriginTransform : sm_lib/Frames and Transforms/Rigid Transform  TranslationMethod=Cartesian  TranslationStandardOffset=0  TranslationLengthUnit=m  TranslationStandardAxis=+Z  TranslationCartesianOffset=[0, 0, 0]  TranslationROffset=0  TranslationROffsetUnits=m  TranslationZOffset=0  TranslationZOffsetUnits=m  TranslationThetaOffset=0  TranslationThetaOffsetUnits=deg  RotationMethod=RotationSequence  RotationAngleUnits=deg  RotationStandardAxis=+Z  RotationAngle=0.0  RotationArbitraryAxis=[0 0 1]  FollAlignAxisA=+X  BaseAlignAxisA=+Y  FollAlignAxisB=+Y  BaseAlignAxisB=+Z  RotationSequenceAxes=BaseAxes  RotationSequence=XYZ  RotationSequenceAngles=[0, 0, 0]  RotationSequenceAnglesUnits=rad  RotationMatrix=[1 0 0; 0 1 0; 0 0 1]
  ReferenceFrame : sm_lib/Frames and Transforms/Reference Frame
  Visual : sm_lib/Body Elements/File Solid  ExtGeomFileName=base.stl  UnitType=Custom  ExtGeomFileUnits=m  StepReaderType=HEX  ExportConvexHullGeometry=off  InertiaType=Custom  Mass=0  MassUnits=kg  CenterOfMass=[0, 0, 0]  CenterOfMassUnits=m  MomentsOfInertia=[0, 0, 0]  MomentsOfInertiaUnits=kg*m^2  ProductsOfInertia=[0, 0, 0]  ProductsOfInertiaUnits=kg*m^2  BasedOnType=DensityFromFile  Density=1000  DensityUnits=kg/m^3  DoExposeReferenceFrame=on  SerializedFrames=<Frames/>  GraphicType=FromGeometry  MarkerShape=Sphere  MarkerSize=10  GraphicVisPropType=SimpleVisualProperties  GraphicDiffuseColor=[0.7, 0.7, 0.7]  GraphicSpecularColor=[0.5 0.5 0.5 1.0]  GraphicAmbientColor=[0.15 0.15 0.15 1.0]  GraphicEmissiveColor=[0.0 0.0 0.0 1.0]  GraphicShininess=75  GraphicOpacity=1
  VisualOriginTransform : sm_lib/Frames and Transforms/Rigid Transform  TranslationMethod=Cartesian  TranslationStandardOffset=0  TranslationLengthUnit=m  TranslationStandardAxis=+Z  TranslationCartesianOffset=[0, 0, 0]  TranslationROffset=0  TranslationROffsetUnits=m  TranslationZOffset=0  TranslationZOffsetUnits=m  TranslationThetaOffset=0  TranslationThetaOffsetUnits=deg  RotationMethod=RotationSequence  RotationAngleUnits=deg  RotationStandardAxis=+Z  RotationAngle=0.0  RotationArbitraryAxis=[0 0 1]  FollAlignAxisA=+X  BaseAlignAxisA=+Y  FollAlignAxisB=+Y  BaseAlignAxisB=+Z  RotationSequenceAxes=BaseAxes  RotationSequence=XYZ  RotationSequenceAngles=[0, 0, 3.141592653589793]  RotationSequenceAnglesUnits=rad  RotationMatrix=[1 0 0; 0 1 0; 0 0 1]
  shoulder_pan_joint_AxisTransform : sm_lib/Frames and Transforms/Rigid Transform  TranslationMethod=Cartesian  TranslationStandardOffset=0  TranslationLengthUnit=m  TranslationStandardAxis=+Z  TranslationCartesianOffset=[0, 0, 0]  TranslationROffset=0  TranslationROffsetUnits=m  TranslationZOffset=0  TranslationZOffsetUnits=m  TranslationThetaOffset=0  TranslationThetaOffsetUnits=deg  RotationMethod=ArbitraryAxis  RotationAngleUnits=rad  RotationStandardAxis=+Z  RotationAngle=0  RotationArbitraryAxis=[1, 0, 0]  FollAlignAxisA=+X  BaseAlignAxisA=+Y  FollAlignAxisB=+Y  BaseAlignAxisB=+Z  RotationSequenceAxes=FollowerAxes  RotationSequence=XYX  RotationSequenceAngles=[0 0 0]  RotationSequenceAnglesUnits=deg  RotationMatrix=[1 0 0; 0 1 0; 0 0 1]
  shoulder_pan_joint_OriginTransform : sm_lib/Frames and Transforms/Rigid Transform  TranslationMethod=Cartesian  TranslationStandardOffset=0  TranslationLengthUnit=m  TranslationStandardAxis=+Z  TranslationCartesianOffset=[0, 0, 0.1519]  TranslationROffset=0  TranslationROffsetUnits=m  TranslationZOffset=0  TranslationZOffsetUnits=m  TranslationThetaOffset=0  TranslationThetaOffsetUnits=deg  RotationMethod=RotationSequence  RotationAngleUnits=deg  RotationStandardAxis=+Z  RotationAngle=0.0  RotationArbitraryAxis=[0 0 1]  FollAlignAxisA=+X  BaseAlignAxisA=+Y  FollAlignAxisB=+Y  BaseAlignAxisB=+Z  RotationSequenceAxes=BaseAxes  RotationSequence=XYZ  RotationSequenceAngles=[0, 0, 0]  RotationSequenceAnglesUnits=rad  RotationMatrix=[1 0 0; 0 1 0; 0 0 1]
  F : PMIOPort  Side=Left
  F1 : PMIOPort  Port=2  Side=Right
  connections:
  Inertia/RConn1 -- InertiaOriginTransform/RConn1
  ReferenceFrame/RConn1 -- InertiaOriginTransform/LConn1 -- VisualOriginTransform/LConn1 -- shoulder_pan_joint_OriginTransform/LConn1 -- F/RConn1
  Visual/RConn1 -- VisualOriginTransform/RConn1
  shoulder_pan_joint_AxisTransform/RConn1 -- F1/RConn1
  shoulder_pan_joint_AxisTransform/LConn1 -- shoulder_pan_joint_OriginTransform/RConn1
